simulink library "solar_pressure_lib"  (R2016b)
settings: Solver=VariableStepAuto  StartTime=0.0  StopTime=10.0  RelTol=1e-3
undefined symbols (not defined in the file or in its folder): sim_params
libraries: aerolibutil x1
settings Model: Creator=bbarz_000  LastModifiedBy=taylorreynolds
settings OptimizationCC: LifeSpan=inf
settings DebuggingCC: SFExecutionAtInitializationDiag=none

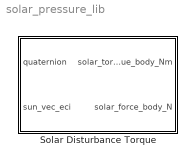
== system solar_pressure_lib ==
  Solar Disturbance Torque : Subsystem

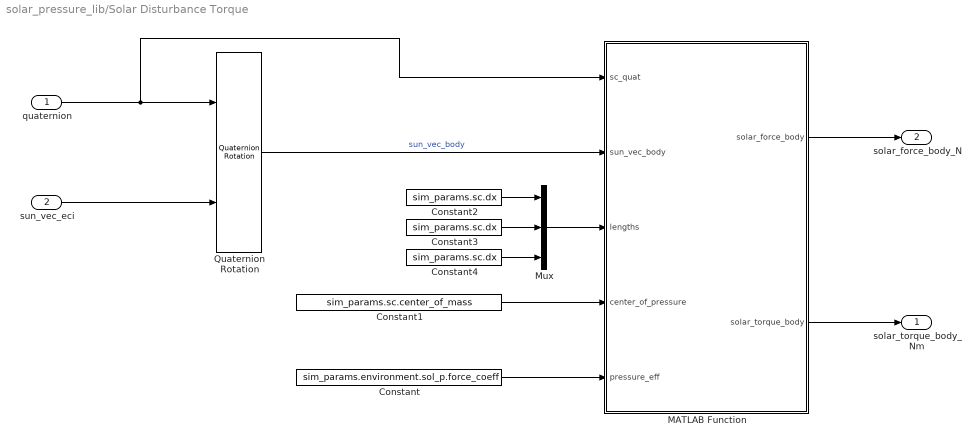
== system solar_pressure_lib/Solar Disturbance Torque ==
  quaternion : Inport
  sun_vec_eci : Inport  Port=2
  Constant : Constant  Value=sim_params.environment.sol_p.force_coeff
  Constant1 : Constant  Value=sim_params.sc.center_of_mass
  Constant2 : Constant  Value=sim_params.sc.dx
  Constant3 : Constant  Value=sim_params.sc.dx
  Constant4 : Constant  Value=sim_params.sc.dx
  MATLAB Function : MATLAB Function  TreatAsAtomicUnit=on
  Mux : Mux  Inputs=3
  Quaternion Rotation : aerolibutil/Quaternion Rotation
  solar_torque_body_Nm : Outport
  solar_force_body_N : Outport  Port=2
  wires:
  quaternion/1 -> MATLAB Function/1(sc_quat), Quaternion Rotation/1
  sun_vec_eci/1 -> Quaternion Rotation/2
  MATLAB Function/2(solar_torque_body) -> solar_torque_body_Nm/1
  Quaternion Rotation/1 -> MATLAB Function/2(sun_vec_body)  "sun_vec_body"
  Constant/1 -> MATLAB Function/5(pressure_eff)
  Constant1/1 -> MATLAB Function/4(center_of_pressure)
  Mux/1 -> MATLAB Function/3(lengths)
  Constant2/1 -> Mux/1
  Constant3/1 -> Mux/2
  Constant4/1 -> Mux/3
  MATLAB Function/1(solar_force_body) -> solar_force_body_N/1

== matlab function solar_pressure_lib/Solar Disturbance Torque/MATLAB Function ==
  data: sc_quat input size=4; solar_force_body output size=3; sun_vec_body input size=3; lengths input size=3; center_of_pressure input size=3; pressure_eff input size=1; solar_torque_body output size=3
function [solar_force_body,solar_torque_body] = solar_force_torque(sc_quat,sun_vec_body,lengths,center_of_pressure,pressure_eff)
%#codegen

% Computes the solar force and solar torque for the s/c given the sun's
% location and the current orientation
%   Ref: dR-D-F, Spacecraft Dynamics & Control, 2013, pp. 228-229

% S/C dimensions accounting for solar panels open
lenx1   = lengths(1);   % dx (top view) is 0.11
lenx2   = lengths(3);  % dx (side view) is 0.3
leny    = lengths(2);   % dy = 0.3
lenz    = lengths(3);   % dz = 0.3

q       = sc_quat;
p       = pressure_eff;
DCM     = my_quat2dcm(q);
CoP = reshape(center_of_pressure, [3 1]);
s_body = reshape(sun_vec_body, [3 1]);

% Make sure its a unit vector
s_body  = s_body/norm(s_body);

% Define std body vectors in body frame
body_vecs = [1 0 0;
            -1 0 0;
            0 1 0;
            0 -1 0;
            0 0 1;
            0 0 -1]';
        
% Rotate body vectors to account for current orientation
rot_body_vecs   = DCM*body_vecs;  

% Compute areas for each face
areas   = [leny*lenz,leny*lenz,lenx2*lenz,lenx2*lenz,lenx1*leny,lenx1*leny];

f = zeros(3,6);
for i = 1:6
    if dot(s_body, rot_body_vecs(:,i)) > 0
        f(:,i) = -p*dot(rot_body_vecs(:,i),s_body)*areas(i)*s_body;
    end
end
solar_force_body = sum(f, 2);
solar_torque_body = cross(CoP,solar_force_body);

end

function DCM = my_quat2dcm( q )
q0  = q(1);
q1  = q(2);
q2  = q(3);
q3  = q(4);

DCM     = [ q0^2+q1^2-q2^2-q3^3  2*q1*q2-2*q0*q3         2*q1*q3+2*q0*q2;
            2*q1*q2+2*q0*q3      q0^2-q1^2+q2^2+q3^2     2*q2*q3-2*q0*q1;
            2*q1*q3-2*q0*q2      2*q2*q3+2*q0*q1         q0^2-q1^2-q2^2+q3^2 ];
end
